simulink model "qError"  (R2018a)
settings: Solver=VariableStepAuto  StartTime=0.0  StopTime=10.0  RelTol=1e-3
settings Model: Creator=henry  LastModifiedBy=henry

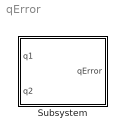
== system qError ==
  Subsystem : Subsystem  mask(Quaternion Error){}
      mask help: This block computes the quaternion error given two input quaternions.

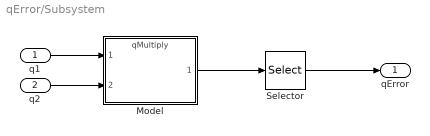
== system qError/Subsystem ==
  q1 : Inport
  q2 : Inport  Port=2
  Model : ModelReference  ModelNameDialog=qMultiply  SimulationMode=Normal  ModelReferenceVersion=1.2
  Selector : Selector  InputPortWidth=4  IndexOptions=Index vector (dialog)  Indices=[1:3]  OutputSizes=1
  qError : Outport
  wires:
  q2/1 -> Model/2
  Selector/1 -> qError/1
  q1/1 -> Model/1
  Model/1 -> Selector/1
